simulink model "Q2_1_1"  (R2023b)
settings: Solver=VariableStepAuto  StartTime=0.0  StopTime=10.0  RelTol=1e-3
settings Model: Creator=sayed  LastModifiedBy=sayed

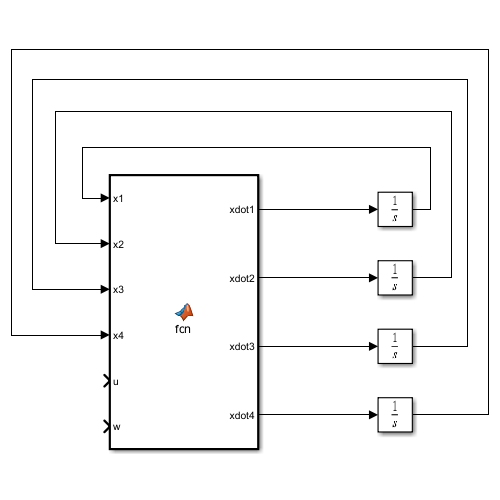
[thumbnail: Simulink's stored preview of the top-level diagram]
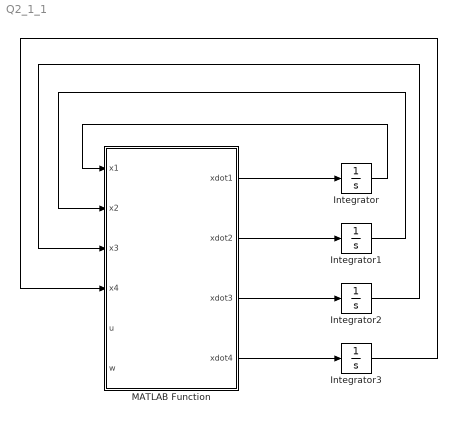
== system Q2_1_1 ==
  Integrator : Integrator
  Integrator1 : Integrator
  Integrator2 : Integrator  InitialCondition=2
  Integrator3 : Integrator  InitialCondition=0.5
  MATLAB Function : MATLAB Function  TreatAsAtomicUnit=on
  wires:
  MATLAB Function/1(xdot1) -> Integrator/1
  MATLAB Function/2(xdot2) -> Integrator1/1
  MATLAB Function/3(xdot3) -> Integrator2/1
  MATLAB Function/4(xdot4) -> Integrator3/1
  Integrator/1 -> MATLAB Function/1(x1)
  Integrator1/1 -> MATLAB Function/2(x2)
  Integrator2/1 -> MATLAB Function/3(x3)
  Integrator3/1 -> MATLAB Function/4(x4)

== matlab function Q2_1_1/MATLAB Function ==
  data: x1 input; x2 input; x3 input; x4 input; u input; xdot1 output; w input; xdot2 output; xdot3 output; xdot4 output
function [xdot1, xdot2, xdot3, xdot4] = fcn(x1, x2, x3, x4, u, w)

% Parameter Values

m1 = 10000;
m2 = 8000;
k = 500000;
c = 5000;

% State-Equations

xdot1 = x3;
xdot2 = x4;
xdot3 = (1 / m1) / (k * (-x1 + x2) + c * (-x3 + x4) + u + w);
xdot4 = (1 / m2) / (k * (x1 - x2) + c * (x3 - x4));
